simulink model "sampleModel1626_5"  (R2023a)
settings: Solver=VariableStepAuto  StartTime=0.0  StopTime=10.0  RelTol=1e-3
libraries: hdlsllib x6
settings Model: Creator=user1  LastModifiedBy=user1

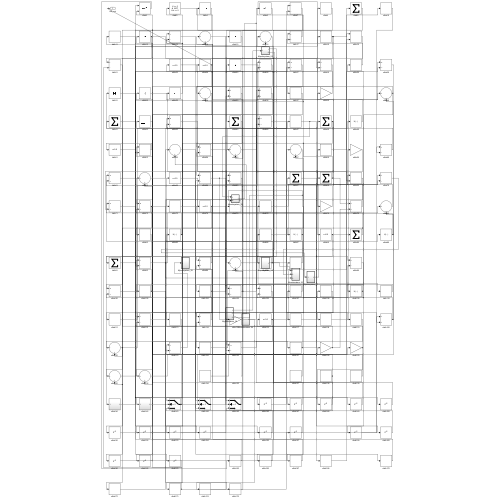
[thumbnail: Simulink's stored preview of the top-level diagram]
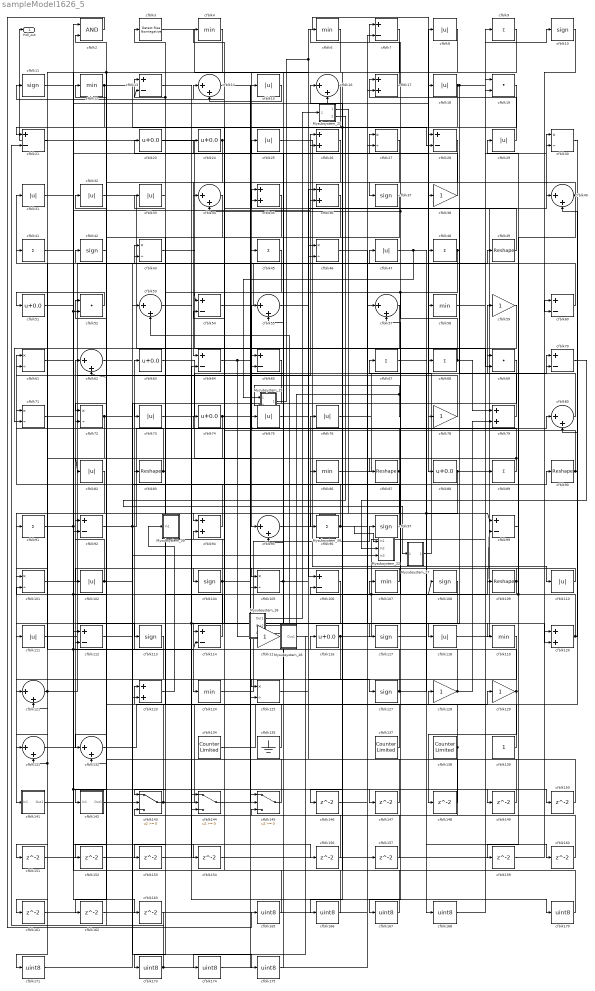
== system sampleModel1626_5 ==
  Mysubsystem_18 : Subsystem  TreatAsAtomicUnit=on  RTWFcnName=Mysubsystem_18
      settings: RTWFcnNameOpts=User specified  RTWFileNameOpts=Use function name
  Mysubsystem_19 : Subsystem  TreatAsAtomicUnit=on  RTWFcnName=Mysubsystem_19
      settings: RTWFcnNameOpts=User specified  RTWFileNameOpts=Use function name
  Mysubsystem_22 : Subsystem  TreatAsAtomicUnit=on  RTWFcnName=Mysubsystem_22
      settings: RTWFcnNameOpts=User specified  RTWFileNameOpts=Use function name
  Mysubsystem_25 : Subsystem  TreatAsAtomicUnit=on  RTWFcnName=Mysubsystem_25
      settings: RTWFcnNameOpts=User specified  RTWFileNameOpts=Use function name
  Mysubsystem_27 : Subsystem  TreatAsAtomicUnit=on  RTWFcnName=Mysubsystem_27
      settings: RTWFcnNameOpts=User specified  RTWFileNameOpts=Use function name
  Mysubsystem_28 : Subsystem  TreatAsAtomicUnit=on  RTWFcnName=Mysubsystem_28
      settings: RTWFcnNameOpts=User specified  RTWFileNameOpts=Use function name
  Mysubsystem_38 : Subsystem  TreatAsAtomicUnit=on  RTWFcnName=Mysubsystem_38
      settings: RTWFcnNameOpts=User specified  RTWFileNameOpts=Use function name
  Mysubsystem_39 : Subsystem  TreatAsAtomicUnit=on  RTWFcnName=Mysubsystem_39
      settings: RTWFcnNameOpts=User specified  RTWFileNameOpts=Use function name
  cfblk{10..11,37,42,97,104,108,113,117,127} (10 alike) : Signum
  cfblk{27,30,43,46,61,71..72,101,105,125} (10 alike) : Product  Inputs=*/  OutDataTypeStr=uint8  RndMeth=Zero  SaturateOnIntegerOverflow=on
  cfblk{8,15,18,25,29,31..33,47,73,75..76,82,102,110..111,118} (17 alike) : Abs  OutDataTypeStr=uint8  SaturateOnIntegerOverflow=off
  cfblk{7,13,21,28,54,60,64..65,70,92,99,106,112,114} (14 alike) : Sum  Inputs=+-  OutDataTypeStr=uint8
  cfblk{4,6,12,58,86,107,119,124} (8 alike) : MinMax  OutDataTypeStr=uint8
  cfblk{49,83,87,90,109} (5 alike) : Reshape
  cfblk{38,59,78,115,128..129} (6 alike) : Gain  OutDataTypeStr=uint8
  cfblk{23..24,51,63,74,88,116} (7 alike) : Bias  Bias=0.0  SaturateOnIntegerOverflow=off
  cfblk{17,26,35..36,79,94,120,123} (8 alike) : Sum  OutDataTypeStr=uint8
  cfblk{14,16,34,40,53,55,57,62,80,95,121,131..132} (13 alike) : Sum  Inputs=|++  OutDataTypeStr=uint8
  cfblk134 : hdlsllib/Sources/Counter Limited  uplimit=7  tsamp=-1
  cfblk135 : Ground
  cfblk137 : hdlsllib/Sources/Counter Limited  uplimit=7  tsamp=-1
  cfblk138 : hdlsllib/Sources/Counter Limited  uplimit=7  tsamp=-1
  cfblk139 : Constant  OutDataTypeStr=uint8  SampleTime=-1
  cfblk141 : Subsystem
      settings: LibrarySourceBlock=|
      | hdlsllib/Ports &
      | Subsystems/Subsystem
  cfblk142 : Subsystem
      settings: LibrarySourceBlock=|
      | hdlsllib/Ports &
      | Subsystems/Subsystem
  cfblk143 : Switch  OutDataTypeStr=uint8  SaturateOnIntegerOverflow=off  InputSameDT=off
  cfblk144 : Switch  OutDataTypeStr=uint8  SaturateOnIntegerOverflow=off  InputSameDT=off
  cfblk145 : Switch  OutDataTypeStr=uint8  SaturateOnIntegerOverflow=off  InputSameDT=off
  cfblk{146..154,156..157,159..163} (16 alike) : Delay  SampleTime=1
  cfblk{165..168,170..171,173..175} (9 alike) : DataTypeConversion  OutDataTypeStr=uint8  SaturateOnIntegerOverflow=off  RndMeth=Floor
  cfblk19 : DotProduct  OutDataTypeStr=uint8
  cfblk2 : Logic  AllPortsSameDT=off  OutDataTypeStr=boolean
  cfblk3 : hdlsllib/Logic and Bit Operations/Detect Rise Nonnegative  vinit=0  OutDataTypeStr=uint8
  cfblk{9,41,45,48,67..68,89,91,96} (9 alike) : Sum  Inputs=+  OutDataTypeStr=uint8
  cfblk52 : DotProduct  OutDataTypeStr=uint8
  cfblk69 : DotProduct  OutDataTypeStr=uint8
  Hdl_out : Outport  OutDataTypeStr=uint8
  wires:
  cfblk107/1 -> cfblk104/1
  cfblk25/1 -> cfblk110/1
  cfblk83/1 -> cfblk61/1, cfblk43/2
  cfblk88/1 -> cfblk141/1(In1), cfblk30/2
  cfblk95/1 -> cfblk76/1
  cfblk121/1 -> cfblk47/1, cfblk161/1
  cfblk47/1 -> Mysubsystem_19/1(In1), cfblk99/1, cfblk160/1
  cfblk124/1 -> cfblk97/1
  cfblk128/1 -> cfblk63/1, cfblk79/2
  cfblk30/1 -> cfblk123/1
  cfblk26/1 -> cfblk64/1
  cfblk68/1 -> cfblk23/1, cfblk34/2, cfblk79/1
  cfblk118/1 -> cfblk30/1
  cfblk16/1 -> cfblk95/1
  cfblk36/1 -> cfblk73/1
  cfblk131/1 -> cfblk62/1
  cfblk90/1 -> cfblk14/1, cfblk40/2
  cfblk21/1 -> cfblk101/1
  cfblk143/1 -> cfblk129/1, cfblk32/1
  cfblk60/1 -> cfblk31/1
  cfblk106/1 -> cfblk124/1
  cfblk12/1 -> cfblk121/1, cfblk28/2
  cfblk46/1 -> cfblk119/1
  cfblk7/1 -> cfblk45/1
  cfblk69/1 -> cfblk123/2
  cfblk111/1 -> cfblk113/1
  cfblk139/1 -> cfblk52/1
  cfblk74/1 -> cfblk145/1, cfblk153/1
  cfblk61/1 -> cfblk27/1
  cfblk78/1 -> cfblk61/2
  cfblk101/1 -> cfblk26/1
  cfblk137/1 -> cfblk13/1
  cfblk94/1 -> cfblk71/1
  cfblk120/1 -> cfblk29/1, cfblk57/2, cfblk80/2
  cfblk134/1 -> cfblk128/1
  cfblk86/1 -> cfblk8/1
  cfblk43/1 -> cfblk78/1
  cfblk54/1 -> cfblk27/2
  cfblk109/1 -> cfblk102/1, cfblk106/2
  cfblk97/1 -> cfblk42/1
  cfblk9/1 -> cfblk96/1
  cfblk13/1 -> cfblk120/2, cfblk147/1
  cfblk58/1 -> cfblk9/1
  cfblk10/1 -> cfblk60/2
  cfblk6/1 -> cfblk125/1
  cfblk132/1 -> cfblk89/1
  cfblk4/1 -> cfblk62/2, cfblk92/2
  cfblk48/1 -> cfblk54/1, cfblk167/1, cfblk118/1
  cfblk87/1 -> cfblk55/1, cfblk4/1, cfblk171/1
  cfblk3/1 -> cfblk106/1
  cfblk116/1 -> cfblk19/2, cfblk99/2, cfblk144/3
  cfblk62/1 -> cfblk48/1
  cfblk33/1 -> cfblk13/2, cfblk3/1
  cfblk91/1 -> cfblk36/2, cfblk149/1
  cfblk42/1 -> cfblk72/1
  cfblk34/1 -> cfblk132/1
  cfblk135/1 -> cfblk72/2
  cfblk31/1 -> cfblk112/1
  cfblk49/1 -> cfblk11/1
  cfblk40/1 -> cfblk37/1, cfblk109/1
  cfblk129/1 -> cfblk41/1, cfblk148/1
  cfblk113/1 -> cfblk132/2
  cfblk45/1 -> cfblk143/1
  cfblk23/1 -> cfblk75/1
  cfblk35/1 -> cfblk142/1(In1)
  cfblk96/1 -> cfblk80/1, cfblk25/1
  cfblk32/1 -> cfblk144/1
  cfblk145/1 -> cfblk24/1
  cfblk144/1 -> cfblk90/1
  cfblk38/1 -> cfblk17/1
  cfblk104/1 -> cfblk33/1, cfblk70/2, cfblk162/1
  cfblk28/1 -> cfblk34/1
  cfblk57/1 -> cfblk71/2
  cfblk92/1 -> Mysubsystem_22/3(In3), cfblk57/1
  cfblk29/1 -> cfblk7/1
  cfblk79/1 -> cfblk59/1
  cfblk11/1 -> cfblk52/2, cfblk163/1
  cfblk119/1 -> cfblk131/2, cfblk151/1
  cfblk115/1 -> cfblk49/1
  cfblk15/1 -> cfblk14/2
  cfblk18/1 -> cfblk10/1, cfblk68/1, cfblk131/1
  cfblk82/1 -> cfblk91/1
  cfblk8/1 -> cfblk21/1
  cfblk37/1 -> cfblk55/2
  cfblk110/1 -> cfblk105/1
  cfblk17/1 -> cfblk6/1
  cfblk142/1(Out1) -> cfblk86/1
  cfblk105/1 -> cfblk35/1, cfblk40/1
  cfblk64/1 -> cfblk125/2, cfblk115/1
  cfblk73/1 -> cfblk15/1
  cfblk102/1 -> cfblk92/1, cfblk156/1
  cfblk71/1 -> cfblk145/2, cfblk154/1
  cfblk76/1 -> cfblk58/1
  cfblk75/1 -> cfblk46/1
  cfblk51/1 -> cfblk18/1
  cfblk63/1 -> cfblk105/2
  cfblk114/1 -> cfblk83/1
  cfblk138/1 -> cfblk145/3, cfblk94/2
  cfblk127/1 -> cfblk69/1, cfblk54/2
  cfblk19/1 -> cfblk114/1, cfblk166/1
  cfblk59/1 -> cfblk87/1
  cfblk55/1 -> cfblk46/2
  cfblk65/1 -> cfblk173/1
  cfblk108/1 -> cfblk121/2
  cfblk80/1 -> cfblk38/1
  cfblk52/1 -> cfblk51/1
  cfblk72/1 -> cfblk111/1, cfblk175/1
  cfblk41/1 -> cfblk28/1
  cfblk89/1 -> cfblk43/1, cfblk82/1
  cfblk141/1(Out1) -> cfblk16/2, cfblk108/1, cfblk114/2
  cfblk117/1 -> cfblk70/1
  cfblk125/1 -> cfblk127/1
  cfblk112/1 -> cfblk107/1
  cfblk27/1 -> cfblk146/1
  cfblk146/1 -> cfblk17/2
  cfblk147/1 -> cfblk101/2
  cfblk148/1 -> cfblk16/1
  cfblk149/1 -> cfblk26/2
  cfblk14/1 -> cfblk150/1
  cfblk150/1 -> cfblk36/1
  cfblk151/1 -> cfblk143/2
  cfblk24/1 -> cfblk152/1, Hdl_out/1
  cfblk152/1 -> cfblk64/2
  cfblk153/1 -> cfblk35/2
  cfblk154/1 -> cfblk120/1
  cfblk156/1 -> cfblk144/2
  cfblk157/1 -> cfblk143/3
  cfblk99/1 -> cfblk159/1
  cfblk159/1 -> cfblk60/1
  cfblk160/1 -> cfblk95/2
  cfblk161/1 -> cfblk7/2
  cfblk162/1 -> cfblk112/2
  cfblk163/1 -> cfblk21/2
  cfblk2/1 -> cfblk165/1
  cfblk165/1 -> cfblk74/1
  cfblk166/1 -> cfblk2/1
  cfblk167/1 -> cfblk2/2
  cfblk67/1 -> cfblk168/1
  cfblk168/1 -> cfblk19/1
  cfblk53/1 -> cfblk170/1
  cfblk170/1 -> cfblk116/1
  cfblk171/1 -> cfblk53/1
  cfblk173/1 -> cfblk157/1, cfblk12/1
  cfblk174/1 -> cfblk65/1
  cfblk175/1 -> cfblk65/2
  Mysubsystem_18/3(Out3) -> Mysubsystem_19/2(U), cfblk117/1
  Mysubsystem_18/2(Out2) -> cfblk53/2
  Mysubsystem_19/1(Out1) -> cfblk88/1, cfblk69/2
  cfblk70/1 -> Mysubsystem_22/2(In2)
  Mysubsystem_18/1(Out1) -> Mysubsystem_25/1(In1)
  Mysubsystem_25/1(Out1) -> cfblk94/1
  Mysubsystem_25/2(Out2) -> Mysubsystem_27/1(In1)
  Mysubsystem_27/1(Out1) -> cfblk67/1
  Mysubsystem_28/1(Out1) -> cfblk174/1
  Mysubsystem_38/1(Out1) -> Mysubsystem_22/1(In1)
  cfblk123/1 -> Mysubsystem_39/1(In1)

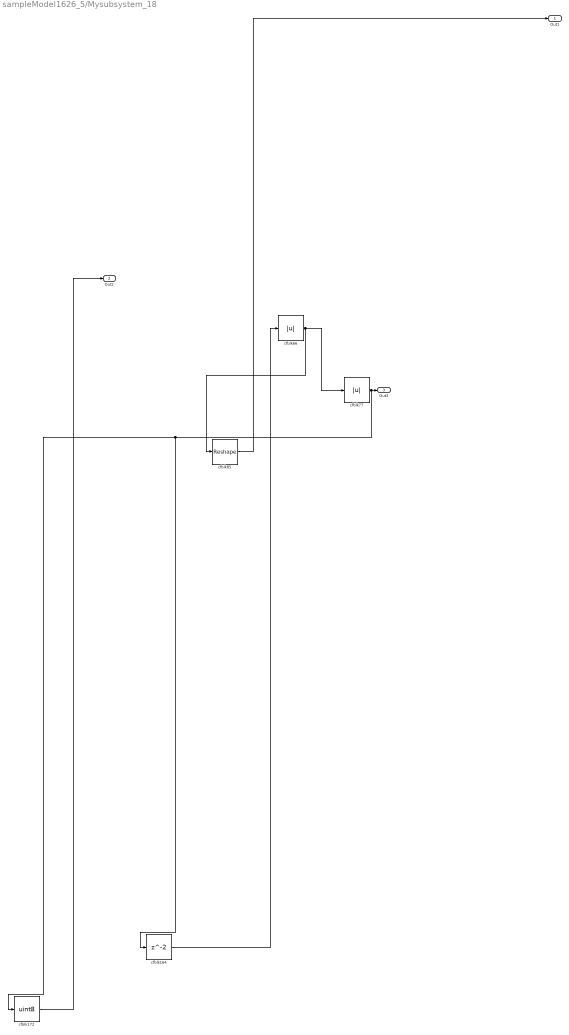
== system sampleModel1626_5/Mysubsystem_18 ==
  cfblk164 : Delay  SampleTime=1
  cfblk172 : DataTypeConversion  OutDataTypeStr=uint8  SaturateOnIntegerOverflow=off  RndMeth=Floor
  cfblk66 : Abs  SaturateOnIntegerOverflow=off
  cfblk77 : Abs  SaturateOnIntegerOverflow=off
  cfblk85 : Reshape
  Out1 : Outport
  Out2 : Outport  Port=2
  Out3 : Outport  Port=3
  wires:
  cfblk172/1 -> Out2/1
  cfblk66/1 -> cfblk85/1, cfblk77/1
  cfblk164/1 -> cfblk66/1
  cfblk77/1 -> cfblk164/1, cfblk172/1, Out3/1
  cfblk85/1 -> Out1/1

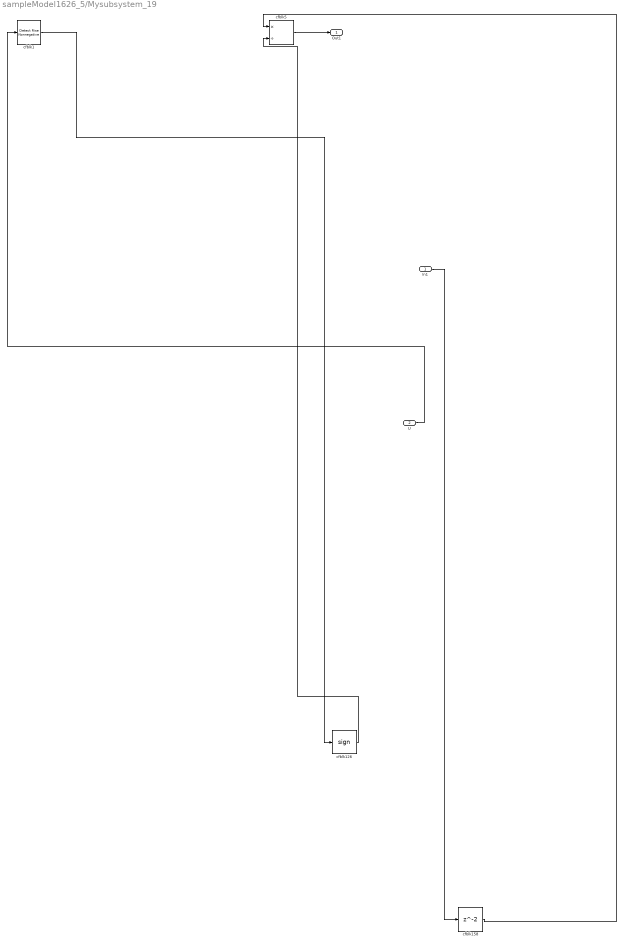
== system sampleModel1626_5/Mysubsystem_19 ==
  In1 : Inport
  U : Inport  Port=2
  cfblk1 : hdlsllib/Logic and Bit Operations/Detect Rise Nonnegative  vinit=0  OutDataTypeStr=boolean
  cfblk126 : Signum
  cfblk158 : Delay  SampleTime=1
  cfblk5 : Product  Inputs=*/  RndMeth=Zero  SaturateOnIntegerOverflow=on
  Out1 : Outport
  wires:
  In1/1 -> cfblk158/1
  cfblk158/1 -> cfblk5/1
  cfblk1/1 -> cfblk126/1
  cfblk126/1 -> cfblk5/2
  U/1 -> cfblk1/1
  cfblk5/1 -> Out1/1

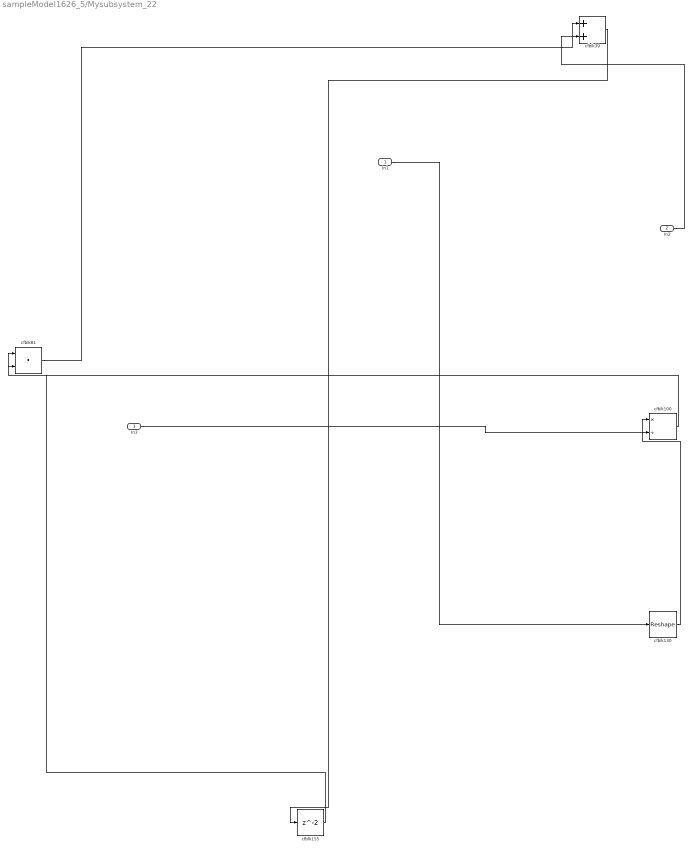
== system sampleModel1626_5/Mysubsystem_22 ==
  In1 : Inport
  In2 : Inport  Port=2
  In3 : Inport  Port=3
  cfblk100 : Product  Inputs=*/  RndMeth=Zero  SaturateOnIntegerOverflow=on
  cfblk130 : Reshape
  cfblk155 : Delay  SampleTime=1
  cfblk39 : Sum
  cfblk81 : DotProduct  OutDataTypeStr=Inherit: Inherit via internal rule
  wires:
  cfblk81/1 -> cfblk39/1
  cfblk130/1 -> cfblk100/1
  cfblk39/1 -> cfblk155/1
  cfblk100/1 -> cfblk81/1
  cfblk155/1 -> cfblk81/2
  In3/1 -> cfblk100/2
  In2/1 -> cfblk39/2
  In1/1 -> cfblk130/1

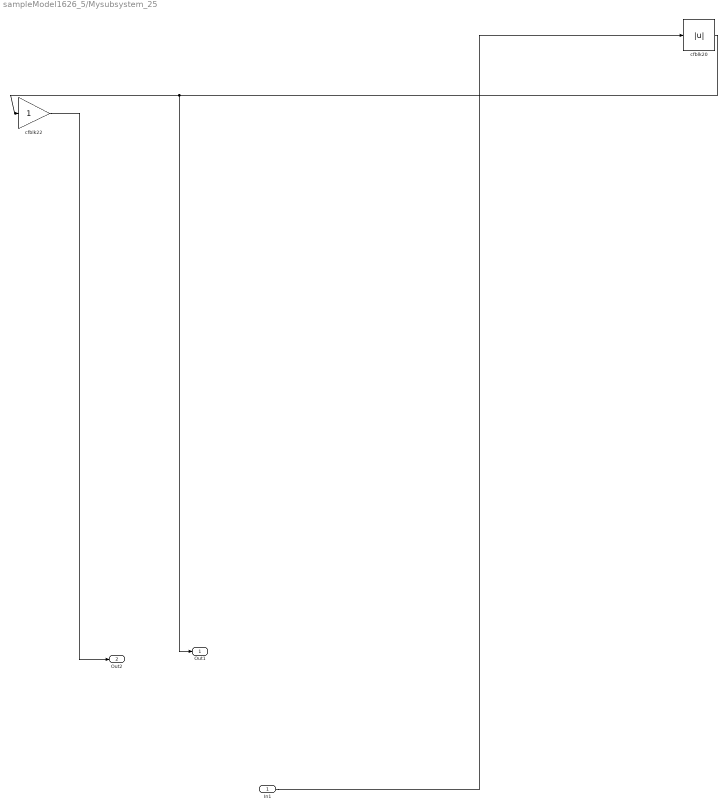
== system sampleModel1626_5/Mysubsystem_25 ==
  In1 : Inport
  cfblk20 : Abs  SaturateOnIntegerOverflow=off
  cfblk22 : Gain
  Out1 : Outport
  Out2 : Outport  Port=2
  wires:
  In1/1 -> cfblk20/1
  cfblk20/1 -> Out1/1, cfblk22/1
  cfblk22/1 -> Out2/1

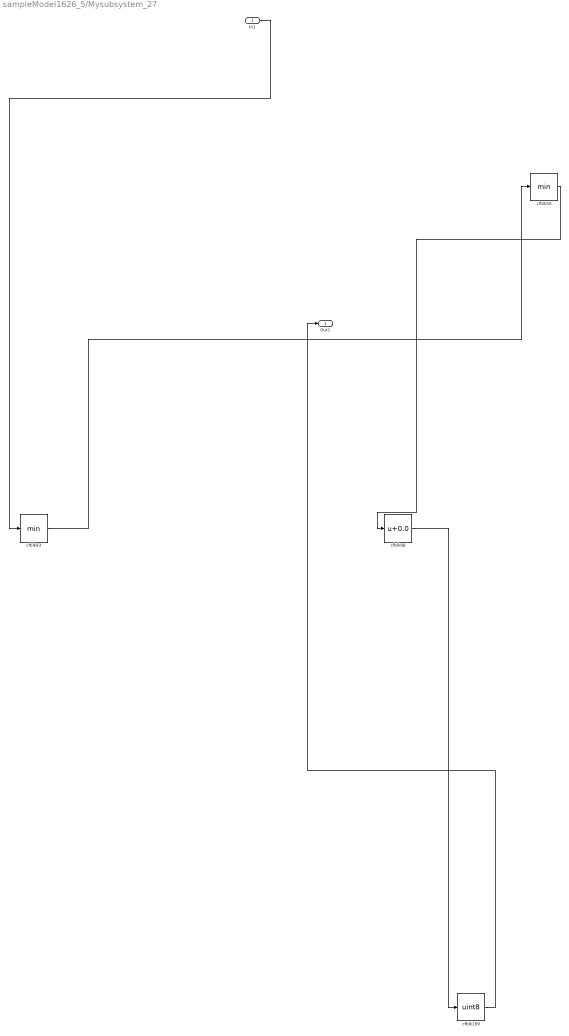
== system sampleModel1626_5/Mysubsystem_27 ==
  In1 : Inport
  cfblk169 : DataTypeConversion  OutDataTypeStr=uint8  SaturateOnIntegerOverflow=off  RndMeth=Floor
  cfblk50 : MinMax
  cfblk93 : MinMax
  cfblk98 : Bias  Bias=0.0  SaturateOnIntegerOverflow=off
  Out1 : Outport
  wires:
  cfblk98/1 -> cfblk169/1
  cfblk50/1 -> cfblk98/1
  cfblk93/1 -> cfblk50/1
  cfblk169/1 -> Out1/1
  In1/1 -> cfblk93/1

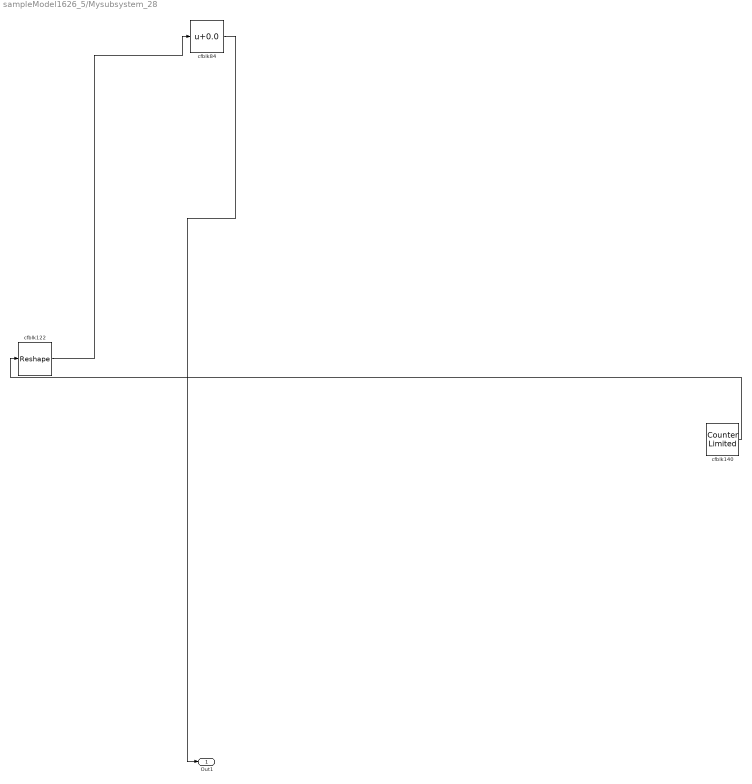
== system sampleModel1626_5/Mysubsystem_28 ==
  cfblk122 : Reshape
  cfblk140 : hdlsllib/Sources/Counter Limited  uplimit=7  tsamp=-1
  cfblk84 : Bias  Bias=0.0  SaturateOnIntegerOverflow=off
  Out1 : Outport
  wires:
  cfblk140/1 -> cfblk122/1
  cfblk84/1 -> Out1/1
  cfblk122/1 -> cfblk84/1

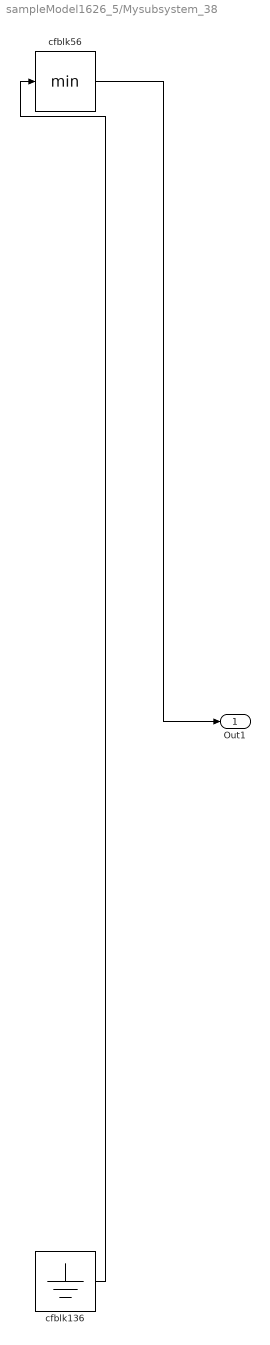
== system sampleModel1626_5/Mysubsystem_38 ==
  cfblk136 : Ground
  cfblk56 : MinMax
  Out1 : Outport
  wires:
  cfblk56/1 -> Out1/1
  cfblk136/1 -> cfblk56/1

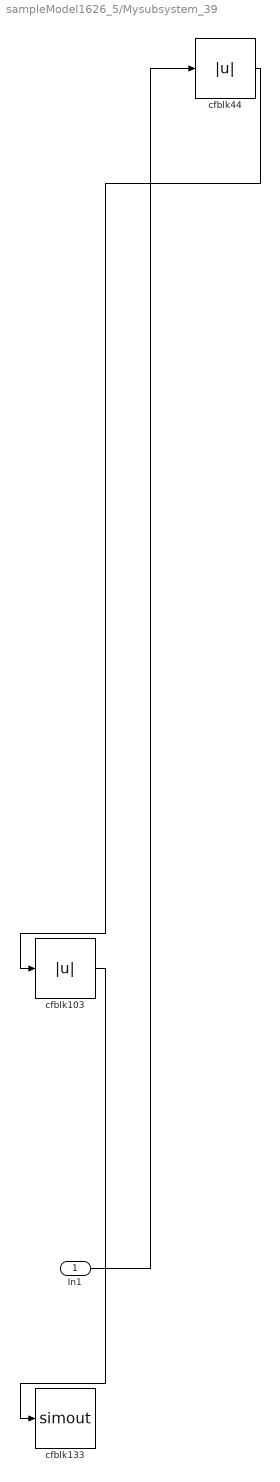
== system sampleModel1626_5/Mysubsystem_39 ==
  In1 : Inport
  cfblk103 : Abs  SaturateOnIntegerOverflow=off
  cfblk133 : ToWorkspace  VariableName=simout  SaveFormat=Timeseries  SampleTime=-1
  cfblk44 : Abs  SaturateOnIntegerOverflow=off
  wires:
  In1/1 -> cfblk44/1
  cfblk44/1 -> cfblk103/1
  cfblk103/1 -> cfblk133/1

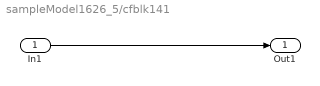
== system sampleModel1626_5/cfblk141 ==
  In1 : Inport
  Out1 : Outport
  wires:
  In1/1 -> Out1/1

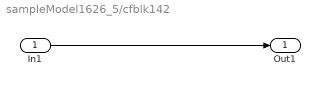
== system sampleModel1626_5/cfblk142 ==
  In1 : Inport
  Out1 : Outport
  wires:
  In1/1 -> Out1/1
